simulink model "mseExecutionSimulations_54"  (R2023b)
settings: Solver=VariableStepAuto  StartTime=0.0  StopTime=10.0  RelTol=1e-3
libraries: simulink x5
settings Model: Creator=iceki  LastModifiedBy=iceki
settings OptimizationCC: ReuseModelBlockBuffer=off

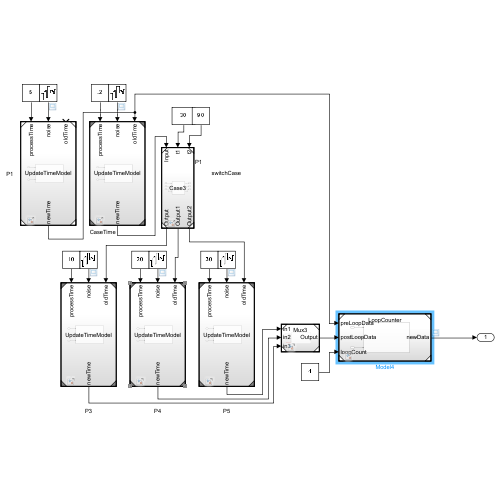
[thumbnail: Simulink's stored preview of the top-level diagram]
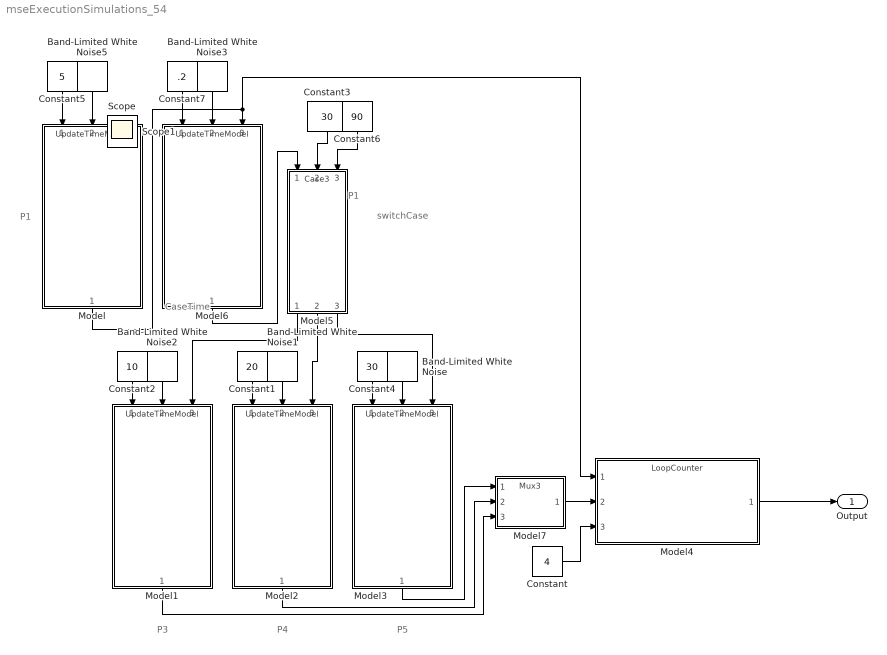
== system mseExecutionSimulations_54 ==
  note: switchCase
  note: CaseTime
  note: P1
  note: P5
  note: P4
  note: P3
  note: P1
  Band-Limited White Noise{,1..3,5} (5 alike) : simulink/Sources/Band-Limited White Noise  Cov=[0.1]  Ts=0.1  seed=[23341]
  Constant : Constant  Value=4
  Constant1 : Constant  Value=20
  Constant2 : Constant  Value=10
  Constant3 : Constant  Value=30
  Constant4 : Constant  Value=30
  Constant5 : Constant  Value=5
  Constant6 : Constant  Value=90
  Constant7 : Constant  Value=.2
  Model{,1..3,6} (5 alike) : ModelReference  ModelNameDialog=UpdateTimeModel.slx  SimulationMode=Normal  ModelReferenceVersion=1.4
  Model4 : ModelReference  ModelNameDialog=LoopCounter.slx  SimulationMode=Normal  ModelReferenceVersion=1.1
  Model5 : ModelReference  ModelNameDialog=Case3.slx  SimulationMode=Normal  ModelReferenceVersion=1.8
  Model7 : ModelReference  ModelNameDialog=Mux3.slx  SimulationMode=Normal  ModelReferenceVersion=1.4
  Output : Outport
  Scope : Scope
  Scope1 : Scope
  wires:
  Constant/1 -> Model4/3
  Constant4/1 -> Model3/1
  Constant1/1 -> Model2/1
  Constant2/1 -> Model1/1
  Constant5/1 -> Model/1
  Band-Limited White Noise/1 -> Model3/2
  Band-Limited White Noise1/1 -> Model2/2
  Band-Limited White Noise2/1 -> Model1/2
  Band-Limited White Noise5/1 -> Model/2
  Model4/1 -> Output/1
  Model5/1 -> Model1/3
  Model5/2 -> Model2/3
  Model5/3 -> Model3/3
  Constant3/1 -> Model5/2
  Constant6/1 -> Model5/3
  Band-Limited White Noise3/1 -> Model6/2
  Constant7/1 -> Model6/1
  Model/1 -> Model6/3, Model4/1
  Model6/1 -> Model5/1
  Model1/1 -> Model7/3
  Model2/1 -> Model7/2
  Model3/1 -> Model7/1
  Model7/1 -> Model4/2
